simulink model "SimulationEchantillinnesClampingMCC_FixedPt"  (R2018b)
settings: Solver=VariableStepAuto  StartTime=0.0  StopTime=2  MaxStep=Ts_elec  RelTol=1e-3
values from neighbouring files (symbols this model uses):
  Cl = 0    [DataMCCEchant.m]
  Imax = Inom    (= 4.4)    [DataMCCEchant.m]
  Imin = 0    [DataMCCEchant.m]
  Kelec = -place(Ae,Be,Pole_elec_desiree)    [DataMCCEchant.m]
  Kmeca = place(Am,Bm,Pole_meca_desiree)    [DataMCCEchant.m]
  Kphi = 0.061    [DataMCCEchant.m]
  Ommax = Omnom    (= 350)    [DataMCCEchant.m]
  Vmax = Vdc    (= 24)    [DataMCCEchant.m]
undefined symbols (not defined in the file or in its folder): DiscIntNeverNeededParam, Ts
libraries: simulink x1
settings Model: Creator=romaindelpoux  LastModifiedBy=Lubin Kerhuel
settings SolverCC: ZeroCrossControl=DisableAll  AlgebraicLoopSolver=LineSearch
settings SFSimCC: SimUseLocalCustomCode=off
settings RTWCC: RTWUseLocalCustomCode=off

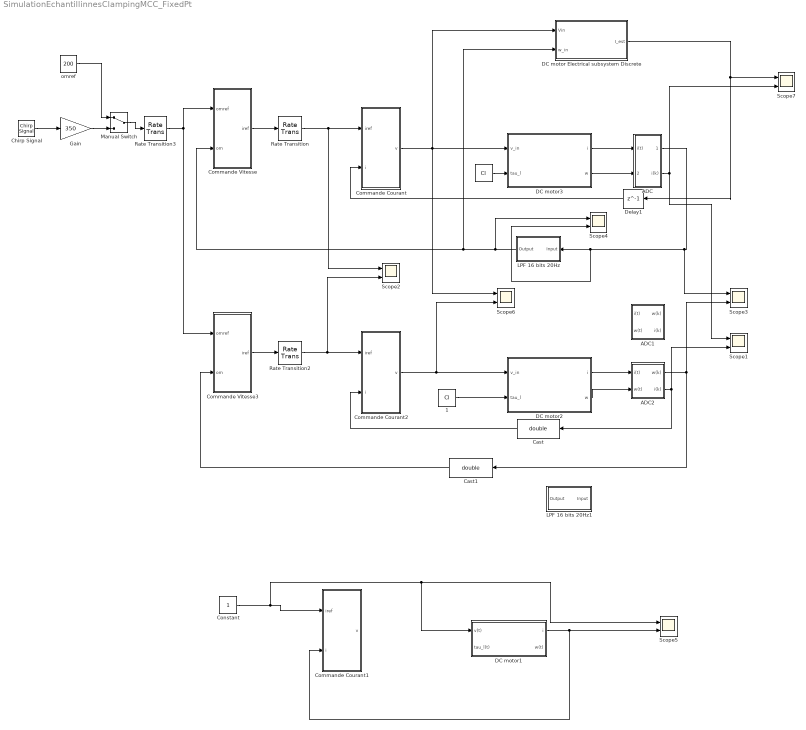
== system SimulationEchantillinnesClampingMCC_FixedPt ==
  " " : Constant  Value=Cl  OutDataTypeStr=Inherit: Inherit via back propagation
  " 1" : Constant  Value=Cl
  ADC : Subsystem
  ADC1 : Subsystem
  ADC2 : Subsystem
  Cast : DataTypeConversion  OutDataTypeStr=double
  Cast1 : DataTypeConversion  OutDataTypeStr=double
  Chirp Signal : simulink/Sources/Chirp Signal  f1=0.1  T=20  f2=5
  Commande Courant : Subsystem
  Commande Courant1 : Subsystem
  Commande Courant2 : Subsystem
  Commande Vitesse : Subsystem
  Commande Vitesse3 : Subsystem
  Constant : Constant
  DC motor Electrical subsystem Discrete : Subsystem
  DC motor1 : Subsystem  mask{R=1.22, L=0.0027, Kphi=0.061, J=0.22e-3, F=.0001, C0=0}
      mask prompts: R "Resistance (R) in Ohms"; L "Inductance (L) in H"; Kphi "Back EMF (Kphi) in V/rad/s"; J "J in kgm²"; F "F in N/rad/s"
      mask DialogControl Container3 Prompt: Electrical Parameters
      mask DialogControl Container3_copy Prompt: Mechanical Parameters
  DC motor2 : Subsystem  mask(Motor PRAVALUX MPM4-0002){R=1.22, L=0.0027, Kphi=0.061, J=0.22e-3, F=.0001, C0=-0.032, mod=0.25}
      mask prompts: R "Resistance (R) in Ohms"; L "Inductance (L) in H"; Kphi "Back EMF (Kphi) in V/rad/s"; J "J in kgm²"; F "F in N/rad/s"; mod "BEMF modulation (default: 0.25, 0 for off)"
      mask help:
      | Continuous time Model for PRAVALUX MPM4 DC motor
      | Caracteristics: 24V DC, 90W, 5.2A, 3000RPM
      |
      | It is a 2nd order model made of two intertwinned system:
      | one 1st order electrical system and one 1st order mechanical system.
      |
      | Modulation on the BEMF can be added to fit with motor current ripple measured
      |
      | Look under mask (Ctrl-U) to see the model
      mask DialogControl Container11 Prompt: Motor
      mask DialogControl Container3 Prompt: Electrical Parameters
      mask DialogControl Container3_copy Prompt: Mechanical Parameters
      mask DialogControl Container14 Prompt: BEMF modulation
      mask Display:
      | color('green');
      | image('MotorPravalux.png');
      | %port_label('input',1,'DC');
      | %port_label('output',1,'BEMF');
  DC motor3 : Subsystem  mask(Motor PRAVALUX MPM4-0002){R=1.22, L=0.0027, Kphi=0.061, J=0.22e-3, F=.0001, C0=-0.032, mod=0.25*0}
      mask prompts: R "Resistance (R) in Ohms"; L "Inductance (L) in H"; Kphi "Back EMF (Kphi) in V/rad/s"; J "J in kgm²"; F "F in N/rad/s"; mod "BEMF modulation (default: 0.25, 0 for off)"
      mask help:
      | Continuous time Model for PRAVALUX MPM4 DC motor
      | Caracteristics: 24V DC, 90W, 5.2A, 3000RPM
      |
      | It is a 2nd order model made of two intertwinned system:
      | one 1st order electrical system and one 1st order mechanical system.
      |
      | Modulation on the BEMF can be added to fit with motor current ripple measured
      |
      | Look under mask (Ctrl-U) to see the model
      mask DialogControl Container11 Prompt: Motor
      mask DialogControl Container3 Prompt: Electrical Parameters
      mask DialogControl Container3_copy Prompt: Mechanical Parameters
      mask DialogControl Container14 Prompt: BEMF modulation
      mask Display:
      | color('green');
      | image('MotorPravalux.png');
      | %port_label('input',1,'DC');
      | %port_label('output',1,'BEMF');
  Delay1 : Delay  DelayLength=1  InitialCondition=0  SampleTime=50e-6
  Gain : Gain  Gain=350  OutDataTypeStr=Inherit: Inherit via back propagation
  LPF 16 bits 20Hz : Subsystem  Tag=FilterWizardSubSystem
      settings: ErrorFcn=dspFilterRealizedInBasicElemsAlgLoopErrFcnCallback
  LPF 16 bits 20Hz1 : Subsystem  Tag=FilterWizardSubSystem
      settings: ErrorFcn=dspFilterRealizedInBasicElemsAlgLoopErrFcnCallback
  Manual Switch : ManualSwitch
  Rate Transition : RateTransition  Deterministic=off  OutPortSampleTime=50e-6
  Rate Transition2 : RateTransition  Deterministic=off  OutPortSampleTime=50e-6
  Rate Transition3 : RateTransition  Deterministic=off  OutPortSampleTime=.002
  Scope{1..7} (7 alike) : Scope  NumInputPorts=2
  omref : Constant  Value=200  OutDataTypeStr=Inherit: Inherit via back propagation
  wires:
  Commande Vitesse/1(iref) -> Rate Transition/1
  DC motor3/1(i) -> ADC/1(i(t))
  DC motor3/2(w) -> ADC/2(w(t))
  ADC/2(i(k)) -> Scope7/2, Scope1/1
  Commande Courant/1(v) -> DC motor Electrical subsystem Discrete/1(Vin), Scope6/1, DC motor3/1(v_in)
  Chirp Signal/1 -> Gain/1
  Rate Transition/1 -> Commande Courant/1(iref), Scope2/1
  DC motor2/2(w) -> ADC2/2(w(t))
  ADC2/2(i(k)) -> Scope1/2, Cast/1
  " 1"/1 -> DC motor2/2(tau_l)
  Commande Vitesse3/1(iref) -> Rate Transition2/1
  Commande Courant2/1(v) -> Scope6/2, DC motor2/1(v_in)
  Rate Transition3/1 -> Commande Vitesse3/1(omref), Commande Vitesse/1(omref)
  Gain/1 -> Manual Switch/2
  Manual Switch/1 -> Rate Transition3/1
  omref/1 -> Manual Switch/1
  ADC/1(w(k)) -> Scope3/1, Scope4/2, LPF 16 bits 20Hz/1(Input)
  Rate Transition2/1 -> Scope2/2, Commande Courant2/1(iref)
  Cast/1 -> Commande Courant2/2(i)
  Cast1/1 -> Commande Vitesse3/2(om)
  LPF 16 bits 20Hz/1(Output) -> Scope4/1, DC motor Electrical subsystem Discrete/2(w_in), Commande Vitesse/2(om)
  ADC2/1(w(k)) -> Cast1/1, Scope3/2
  Constant/1 -> DC motor1/1(v(t)), Scope5/1, Commande Courant1/1(iref)
  DC motor1/1(i) -> Scope5/2, Commande Courant1/2(i)
  " "/1 -> DC motor3/2(tau_l)
  DC motor2/1(i) -> ADC2/1(i(t))
  Delay1/1 -> Commande Courant/2(i)
  DC motor Electrical subsystem Discrete/1(I_est) -> Delay1/1, Scope7/1

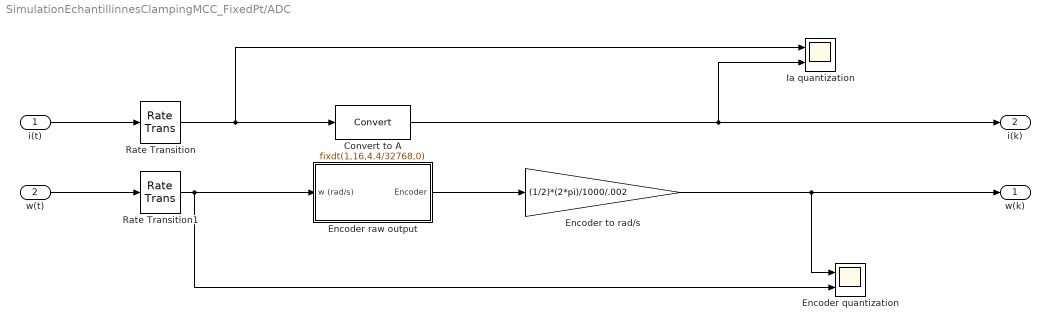
== system SimulationEchantillinnesClampingMCC_FixedPt/ADC ==
  i(t) : Inport
  w(t) : Inport  Port=2
  Convert to A : DataTypeConversion  OutDataTypeStr=fixdt(1,16,4.4/32768,0)  SaturateOnIntegerOverflow=on  LockScale=on
  Encoder quantization : Scope  NumInputPorts=2
  Encoder raw output : Subsystem
  Encoder to rad/s : Gain  Gain=(1/2)*(2*pi)/1000/.002  OutMax=Ommax  OutDataTypeStr=fixdt(1,16)  LockScale=on
  Ia quantization : Scope  NumInputPorts=2
  Rate Transition : RateTransition  Deterministic=off  OutPortSampleTime=.00005
  Rate Transition1 : RateTransition  Deterministic=off  OutPortSampleTime=.002
  w(k) : Outport
  i(k) : Outport  Port=2
  wires:
  Rate Transition/1 -> Ia quantization/1, Convert to A/1
  i(t)/1 -> Rate Transition/1
  w(t)/1 -> Rate Transition1/1
  Encoder to rad/s/1 -> w(k)/1, Encoder quantization/1
  Convert to A/1 -> Ia quantization/2, i(k)/1
  Rate Transition1/1 -> Encoder raw output/1(w (rad/s)), Encoder quantization/2
  Encoder raw output/1(Encoder) -> Encoder to rad/s/1

== system SimulationEchantillinnesClampingMCC_FixedPt/ADC1 ==
  i(t) : Inport
  w(t) : Inport  Port=2
  Rate Transition : RateTransition  Deterministic=off  OutPortSampleTime=50e-6
  Rate Transition1 : RateTransition  Deterministic=off  OutPortSampleTime=.002
  w(k) : Outport
  i(k) : Outport  Port=2
  wires:
  w(t)/1 -> Rate Transition1/1
  i(t)/1 -> Rate Transition/1
  Rate Transition1/1 -> w(k)/1
  Rate Transition/1 -> i(k)/1

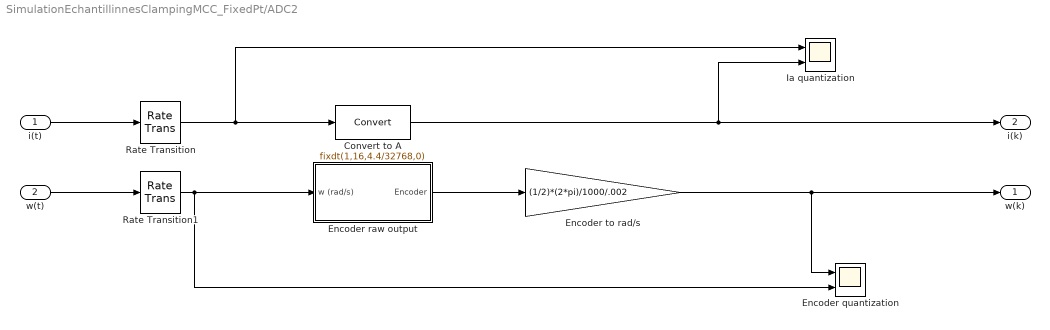
== system SimulationEchantillinnesClampingMCC_FixedPt/ADC2 ==
  i(t) : Inport
  w(t) : Inport  Port=2
  Convert to A : DataTypeConversion  OutDataTypeStr=fixdt(1,16,4.4/32768,0)  SaturateOnIntegerOverflow=on  LockScale=on
  Encoder quantization : Scope  NumInputPorts=2
  Encoder raw output : Subsystem
  Encoder to rad/s : Gain  Gain=(1/2)*(2*pi)/1000/.002  OutMax=Ommax  OutDataTypeStr=fixdt(1,16)  LockScale=on
  Ia quantization : Scope  NumInputPorts=2
  Rate Transition : RateTransition  Deterministic=off  OutPortSampleTime=.00005
  Rate Transition1 : RateTransition  Deterministic=off  OutPortSampleTime=.002
  w(k) : Outport
  i(k) : Outport  Port=2
  wires:
  Encoder raw output/1(Encoder) -> Encoder to rad/s/1
  Rate Transition1/1 -> Encoder quantization/2, Encoder raw output/1(w (rad/s))
  Convert to A/1 -> i(k)/1, Ia quantization/2
  Encoder to rad/s/1 -> Encoder quantization/1, w(k)/1
  w(t)/1 -> Rate Transition1/1
  i(t)/1 -> Rate Transition/1
  Rate Transition/1 -> Convert to A/1, Ia quantization/1

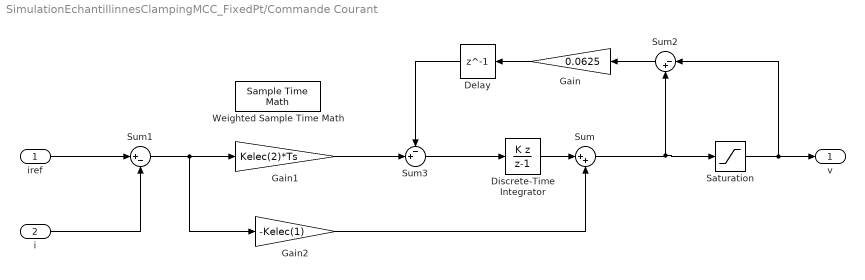
== system SimulationEchantillinnesClampingMCC_FixedPt/Commande Courant ==
  iref : Inport
  i : Inport  Port=2
  Delay : Delay  DelayLength=1  InitialCondition=0
  Discrete-Time Integrator : DiscreteIntegrator  IntegratorMethod=Accumulation: Backward Euler  SampleTime=.00005  OutMax=Vmax*2  OutDataTypeStr=fixdt(1,32)  SaturateOnIntegerOverflow=on  ICPrevOutput=DiscIntNeverNeededParam  ICPrevScaledInput=DiscIntNeverNeededParam
  Gain : Gain  Gain=0.0625  OutDataTypeStr=Inherit: Inherit via back propagation  SaturateOnIntegerOverflow=on
  Gain1 : Gain  Gain=Kelec(2)*Ts  OutMax=2*Imax*Kelec(2)*Ts  OutDataTypeStr=fixdt(1,16)  SaturateOnIntegerOverflow=on
  Gain2 : Gain  Gain=-Kelec(1)  OutMax=Vmax  OutDataTypeStr=fixdt(1,16)  SaturateOnIntegerOverflow=on
  Saturation : Saturate  UpperLimit=Vmax  LowerLimit=-Vmax
  Sum : Sum  Inputs=|++  OutMax=Vmax*2  OutDataTypeStr=fixdt(1,16)  SaturateOnIntegerOverflow=on
  Sum1 : Sum  Inputs=|+-  OutDataTypeStr=fixdt(1,16,12)  SaturateOnIntegerOverflow=on
  Sum2 : Sum  Inputs=|-+  OutDataTypeStr=Inherit: Same as first input
  Sum3 : Sum  Inputs=-+|  OutDataTypeStr=Inherit: Same as accumulator  SaturateOnIntegerOverflow=on  InputSameDT=on
  Weighted Sample Time Math : SampleTimeMath  TsampMathOp=*  weightValue=Kelec(2)  TsampMathImp=Offline Scaling Adjustment
  v : Outport
  wires:
  iref/1 -> Sum1/1
  i/1 -> Sum1/2
  Sum1/1 -> Gain1/1, Gain2/1
  Gain1/1 -> Sum3/2
  Gain2/1 -> Sum/2
  Sum/1 -> Saturation/1, Sum2/2
  Saturation/1 -> v/1, Sum2/1
  Discrete-Time Integrator/1 -> Sum/1
  Sum3/1 -> Discrete-Time Integrator/1
  Sum2/1 -> Gain/1
  Gain/1 -> Delay/1
  Delay/1 -> Sum3/1

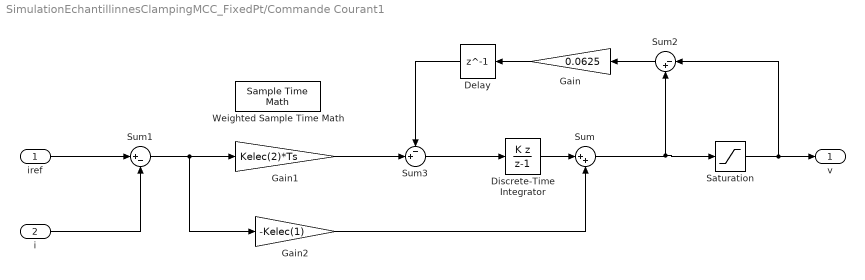
== system SimulationEchantillinnesClampingMCC_FixedPt/Commande Courant1 ==
  iref : Inport
  i : Inport  Port=2
  Delay : Delay  DelayLength=1  InitialCondition=0
  Discrete-Time Integrator : DiscreteIntegrator  IntegratorMethod=Accumulation: Backward Euler  SampleTime=.00005  OutMax=Vmax*2  OutDataTypeStr=fixdt(1,32)  SaturateOnIntegerOverflow=on  ICPrevOutput=DiscIntNeverNeededParam  ICPrevScaledInput=DiscIntNeverNeededParam
  Gain : Gain  Gain=0.0625  OutDataTypeStr=Inherit: Inherit via back propagation  SaturateOnIntegerOverflow=on
  Gain1 : Gain  Gain=Kelec(2)*Ts  OutMax=2*Imax*Kelec(2)*Ts  OutDataTypeStr=fixdt(1,16)  SaturateOnIntegerOverflow=on
  Gain2 : Gain  Gain=-Kelec(1)  OutMax=Vmax  OutDataTypeStr=fixdt(1,16)  SaturateOnIntegerOverflow=on
  Saturation : Saturate  UpperLimit=Vmax  LowerLimit=-Vmax
  Sum : Sum  Inputs=|++  OutMax=Vmax*2  OutDataTypeStr=fixdt(1,16)  SaturateOnIntegerOverflow=on
  Sum1 : Sum  Inputs=|+-  OutDataTypeStr=fixdt(1,16,12)  SaturateOnIntegerOverflow=on
  Sum2 : Sum  Inputs=|-+  OutDataTypeStr=Inherit: Same as first input
  Sum3 : Sum  Inputs=-+|  OutDataTypeStr=Inherit: Same as accumulator  SaturateOnIntegerOverflow=on  InputSameDT=on
  Weighted Sample Time Math : SampleTimeMath  TsampMathOp=*  weightValue=Kelec(2)  TsampMathImp=Offline Scaling Adjustment
  v : Outport
  wires:
  Delay/1 -> Sum3/1
  Gain/1 -> Delay/1
  Sum2/1 -> Gain/1
  Sum3/1 -> Discrete-Time Integrator/1
  Discrete-Time Integrator/1 -> Sum/1
  Saturation/1 -> Sum2/1, v/1
  Sum/1 -> Sum2/2, Saturation/1
  Gain2/1 -> Sum/2
  Gain1/1 -> Sum3/2
  Sum1/1 -> Gain2/1, Gain1/1
  i/1 -> Sum1/2
  iref/1 -> Sum1/1

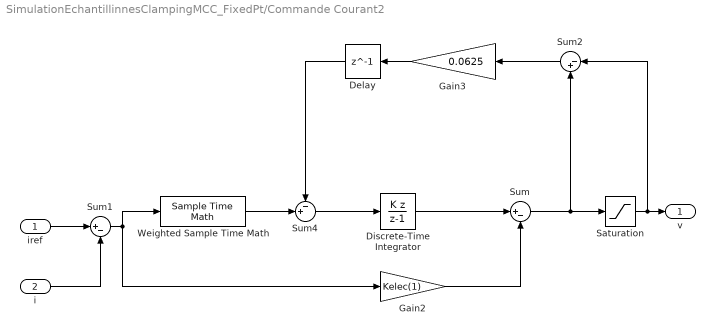
== system SimulationEchantillinnesClampingMCC_FixedPt/Commande Courant2 ==
  iref : Inport
  i : Inport  Port=2
  Delay : Delay  DelayLength=1  InitialCondition=0
  Discrete-Time Integrator : DiscreteIntegrator  IntegratorMethod=Accumulation: Backward Euler  SampleTime=-1  ICPrevOutput=DiscIntNeverNeededParam  ICPrevScaledInput=DiscIntNeverNeededParam
  Gain2 : Gain  Gain=Kelec(1)
  Gain3 : Gain  Gain=0.0625
  Saturation : Saturate  UpperLimit=Vmax  LowerLimit=-Vmax
  Sum : Sum  Inputs=|+-
  Sum1 : Sum  Inputs=|+-
  Sum2 : Sum  Inputs=|-+  OutDataTypeStr=Inherit: Same as accumulator
  Sum4 : Sum  Inputs=-+|
  Weighted Sample Time Math : SampleTimeMath  TsampMathOp=*  weightValue=Kelec(2)  TsampMathImp=Offline Scaling Adjustment
  v : Outport
  wires:
  Weighted Sample Time Math/1 -> Sum4/2
  Sum2/1 -> Gain3/1
  Discrete-Time Integrator/1 -> Sum/1
  Delay/1 -> Sum4/1
  Gain3/1 -> Delay/1
  Sum4/1 -> Discrete-Time Integrator/1
  Sum1/1 -> Weighted Sample Time Math/1, Gain2/1
  Gain2/1 -> Sum/2
  i/1 -> Sum1/2
  iref/1 -> Sum1/1
  Sum/1 -> Sum2/2, Saturation/1
  Saturation/1 -> Sum2/1, v/1

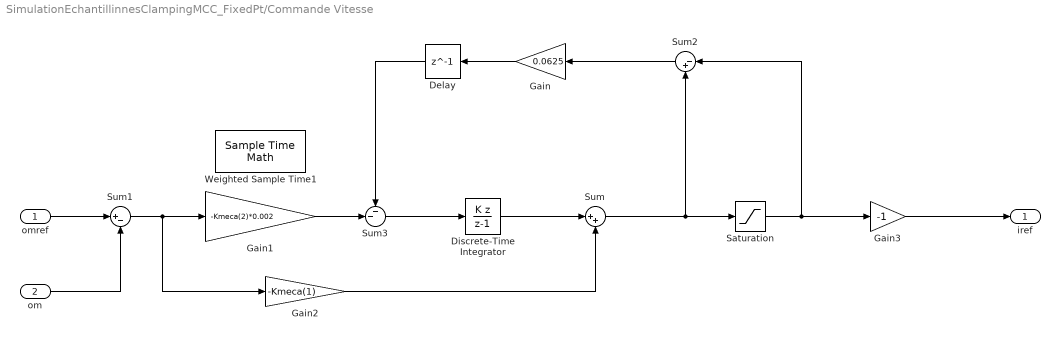
== system SimulationEchantillinnesClampingMCC_FixedPt/Commande Vitesse ==
  omref : Inport  OutMax=[Ommax]  OutDataTypeStr=fixdt(1,16)
  om : Inport  Port=2
  Delay : Delay  DelayLength=1  InitialCondition=0
  Discrete-Time Integrator : DiscreteIntegrator  IntegratorMethod=Accumulation: Backward Euler  SampleTime=.002  OutMin=0  OutMax=Imax*2  OutDataTypeStr=fixdt(1,32)  SaturateOnIntegerOverflow=on  ICPrevOutput=DiscIntNeverNeededParam  ICPrevScaledInput=DiscIntNeverNeededParam
  Gain : Gain  Gain=0.0625  OutDataTypeStr=Inherit: Inherit via back propagation  SaturateOnIntegerOverflow=on
  Gain1 : Gain  Gain=-Kmeca(2)*0.002  OutMin=0  OutMax=abs(Ommax * Kmeca(2) * 0.002)  OutDataTypeStr=fixdt(1,16)
  Gain2 : Gain  Gain=-Kmeca(1)  OutMin=Imin*2  OutMax=Imax*2  OutDataTypeStr=fixdt(1,16)  SaturateOnIntegerOverflow=on
  Gain3 : Gain  Gain=-1  OutMin=Imin  OutMax=Imax  SaturateOnIntegerOverflow=on  OutDataTypeStr=Inherit: Same as input
  Saturation : Saturate  UpperLimit=Imax  LowerLimit=-Imax
  Sum : Sum  Inputs=|++  OutMin=Imin  OutMax=Imax*2  OutDataTypeStr=fixdt(1,16)  SaturateOnIntegerOverflow=on
  Sum1 : Sum  Inputs=|+-  OutMin=-Ommax*2  OutMax=Ommax*2  OutDataTypeStr=fixdt(1,16)
  Sum2 : Sum  Inputs=|-+  OutDataTypeStr=Inherit: Same as accumulator
  Sum3 : Sum  Inputs=--|  OutDataTypeStr=Inherit: Same as accumulator  SaturateOnIntegerOverflow=on  InputSameDT=on
  Weighted Sample Time1 : SampleTimeMath  TsampMathOp=*  weightValue=-Kmeca(2)  TsampMathImp=Offline Scaling Adjustment
  iref : Outport
  wires:
  omref/1 -> Sum1/1
  Gain2/1 -> Sum/2
  om/1 -> Sum1/2
  Sum/1 -> Sum2/2, Saturation/1
  Saturation/1 -> Sum2/1, Gain3/1
  Sum3/1 -> Discrete-Time Integrator/1
  Sum2/1 -> Gain/1
  Gain3/1 -> iref/1
  Sum1/1 -> Gain1/1, Gain2/1
  Gain/1 -> Delay/1
  Delay/1 -> Sum3/1
  Discrete-Time Integrator/1 -> Sum/1
  Gain1/1 -> Sum3/2

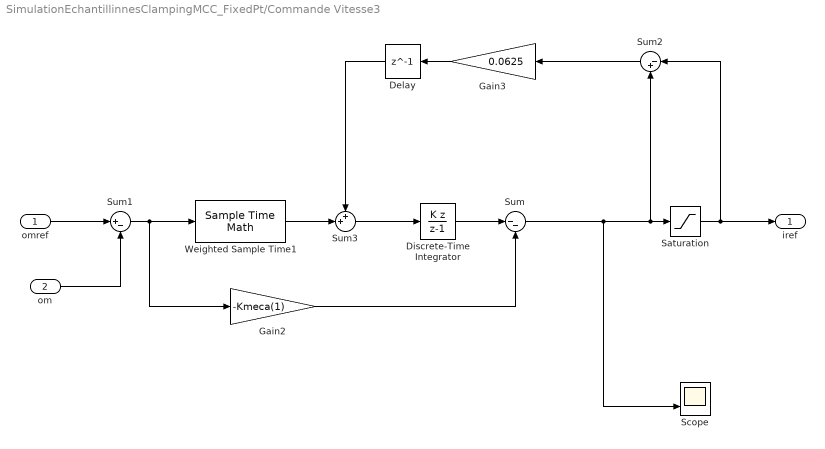
== system SimulationEchantillinnesClampingMCC_FixedPt/Commande Vitesse3 ==
  omref : Inport
  om : Inport  Port=2
  Delay : Delay  DelayLength=1  InitialCondition=0
  Discrete-Time Integrator : DiscreteIntegrator  IntegratorMethod=Accumulation: Backward Euler  SampleTime=-1  ICPrevOutput=DiscIntNeverNeededParam  ICPrevScaledInput=DiscIntNeverNeededParam
  Gain2 : Gain  Gain=-Kmeca(1)
  Gain3 : Gain  Gain=0.0625  OutDataTypeStr=Inherit: Inherit via back propagation
  Saturation : Saturate  UpperLimit=Imax  LowerLimit=-Imax
  Scope : Scope  NumInputPorts=2
  Sum : Sum  Inputs=|--
  Sum1 : Sum  Inputs=|+-
  Sum2 : Sum  Inputs=|-+  OutDataTypeStr=Inherit: Same as accumulator
  Sum3 : Sum  Inputs=++|
  Weighted Sample Time1 : SampleTimeMath  TsampMathOp=*  weightValue=Kmeca(2)
  iref : Outport
  wires:
  Gain2/1 -> Sum/2
  Sum2/1 -> Gain3/1
  Sum1/1 -> Weighted Sample Time1/1, Gain2/1
  omref/1 -> Sum1/1
  om/1 -> Sum1/2
  Sum/1 -> Saturation/1, Sum2/2, Scope/2
  Saturation/1 -> Sum2/1, iref/1
  Discrete-Time Integrator/1 -> Sum/1
  Sum3/1 -> Discrete-Time Integrator/1
  Weighted Sample Time1/1 -> Sum3/2
  Gain3/1 -> Delay/1
  Delay/1 -> Sum3/1

== system SimulationEchantillinnesClampingMCC_FixedPt/DC motor Electrical subsystem Discrete ==
  note: Discrete model of Electrical system:
      | sys_elec = tf(1/R,[L/R 1]);
      | sys_elecz = c2d(sys_elec,50e-6,'zoh')
      |
      | To be used as internal model
  Vin : Inport
  w_in : Inport  Port=2
  Delay : Delay  DelayLength=1  InitialCondition=0  SampleTime=50e-6
  Gain1 : Gain  Gain=-0.977  OutDataTypeStr=fixdt(1,32,9)  SaturateOnIntegerOverflow=on
  Gain3 : Gain  Gain=0.0183  OutMin=[-8.8]  OutMax=8.8  OutDataTypeStr=fixdt(1,16)  SaturateOnIntegerOverflow=on
  Gain4 : Gain  Gain=Kphi  OutDataTypeStr=Inherit: Inherit via back propagation  SaturateOnIntegerOverflow=on
  Rate Transition1 : RateTransition  Deterministic=off  OutPortSampleTime=50e-6
  Sum2 : Sum  Inputs=+--  SaturateOnIntegerOverflow=on
  I_est : Outport
  wires:
  Gain3/1 -> I_est/1
  w_in/1 -> Rate Transition1/1
  Sum2/1 -> Delay/1, Gain3/1
  Gain4/1 -> Sum2/2
  Gain1/1 -> Sum2/3
  Rate Transition1/1 -> Gain4/1
  Vin/1 -> Sum2/1
  Delay/1 -> Gain1/1

== system SimulationEchantillinnesClampingMCC_FixedPt/DC motor1 ==
  v(t) : Inport
  tau_l(t) : Inport  Port=2
  Equation Electrique : Subsystem
  Equation Mecanique : Subsystem
  Gain1 : Gain  Gain=Kphi
  "Gain3  " : Gain  Gain=Kphi
  i : Outport
  w(t) : Outport  Port=2
  wires:
  Gain1/1 -> Equation Mecanique/1(C)
  tau_l(t)/1 -> Equation Mecanique/2(Cl)
  Equation Electrique/1(i(t)) -> i/1, Gain1/1
  Equation Mecanique/1(omega) -> w(t)/1, "Gain3  "/1
  v(t)/1 -> Equation Electrique/1(v)

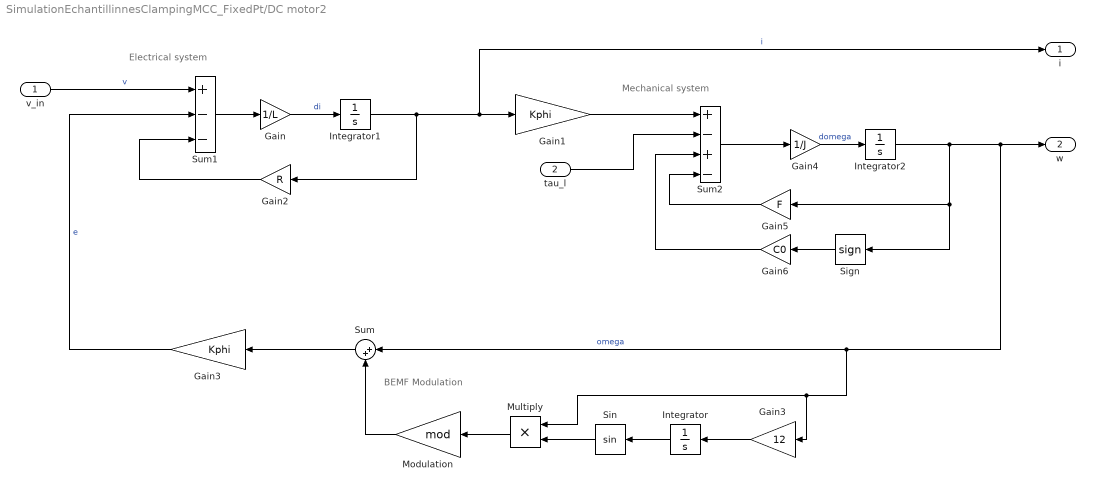
== system SimulationEchantillinnesClampingMCC_FixedPt/DC motor2 ==
  note: BEMF Modulation
  note: Mechanical system
  note: Electrical system
  v_in : Inport  SampleTime=0
  tau_l : Inport  Port=2
  Gain : Gain  Gain=1/L
  Gain1 : Gain  Gain=Kphi
  Gain2 : Gain  Gain=R
  Gain3 : Gain  Gain=12
  "Gain3  " : Gain  Gain=Kphi
  Gain4 : Gain  Gain=1/J
  Gain5 : Gain  Gain=F
  Gain6 : Gain  Gain=C0
  Integrator : Integrator  WrapState=on
  Integrator1 : Integrator
  Integrator2 : Integrator
  Modulation : Gain  Gain=mod
  Multiply : Product
  Sign : Signum
  Sin : Trigonometry
  Sum : Sum  Inputs=|++
  Sum1 : Sum  Inputs=+--
  Sum2 : Sum  Inputs=+-+-
  i : Outport
  w : Outport  Port=2
  wires:
  Sin/1 -> Multiply/2
  Sum/1 -> "Gain3  "/1
  Modulation/1 -> Sum/2
  Multiply/1 -> Modulation/1
  Integrator/1 -> Sin/1
  Gain3/1 -> Integrator/1
  Sum1/1 -> Gain/1
  Gain/1 -> Integrator1/1  "di"
  Integrator1/1 -> Gain2/1, i/1, Gain1/1  "i"
  v_in/1 -> Sum1/1  "v"
  Gain2/1 -> Sum1/3
  "Gain3  "/1 -> Sum1/2  "e"
  tau_l/1 -> Sum2/2
  Gain6/1 -> Sum2/3
  Sign/1 -> Gain6/1
  Integrator2/1 -> w/1, Sum/1, Gain3/1, Multiply/1, Sign/1, Gain5/1  "omega"
  Gain5/1 -> Sum2/4
  Sum2/1 -> Gain4/1
  Gain4/1 -> Integrator2/1  "domega"
  Gain1/1 -> Sum2/1

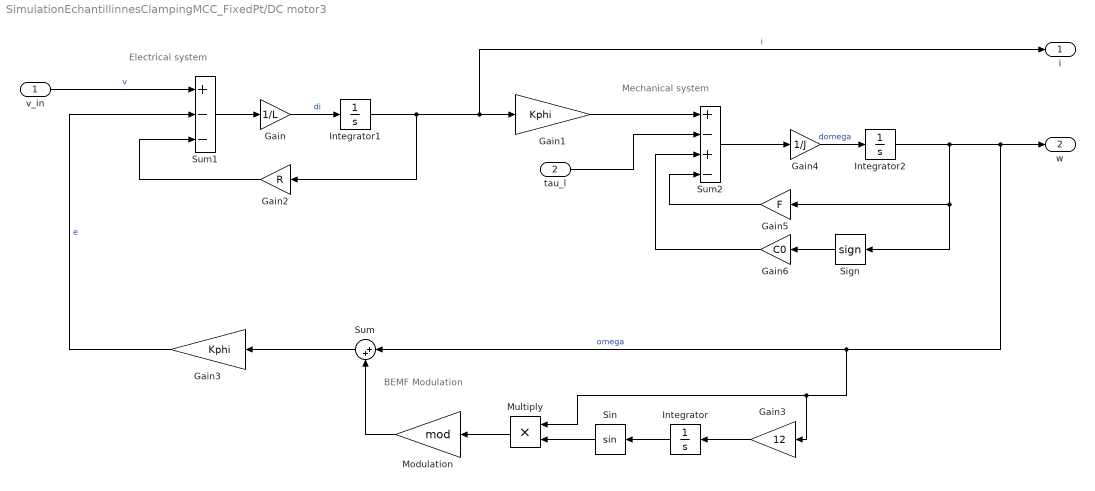
== system SimulationEchantillinnesClampingMCC_FixedPt/DC motor3 ==
  note: Electrical system
  note: Mechanical system
  note: BEMF Modulation
  v_in : Inport  SampleTime=0
  tau_l : Inport  Port=2
  Gain : Gain  Gain=1/L
  Gain1 : Gain  Gain=Kphi
  Gain2 : Gain  Gain=R
  Gain3 : Gain  Gain=12
  "Gain3  " : Gain  Gain=Kphi
  Gain4 : Gain  Gain=1/J
  Gain5 : Gain  Gain=F
  Gain6 : Gain  Gain=C0
  Integrator : Integrator  WrapState=on
  Integrator1 : Integrator
  Integrator2 : Integrator
  Modulation : Gain  Gain=mod
  Multiply : Product
  Sign : Signum
  Sin : Trigonometry
  Sum : Sum  Inputs=|++
  Sum1 : Sum  Inputs=+--
  Sum2 : Sum  Inputs=+-+-
  i : Outport
  w : Outport  Port=2
  wires:
  Gain1/1 -> Sum2/1
  Gain4/1 -> Integrator2/1  "domega"
  Sum2/1 -> Gain4/1
  Gain5/1 -> Sum2/4
  Integrator2/1 -> Gain5/1, Sign/1, Multiply/1, Gain3/1, Sum/1, w/1  "omega"
  Sign/1 -> Gain6/1
  Gain6/1 -> Sum2/3
  tau_l/1 -> Sum2/2
  "Gain3  "/1 -> Sum1/2  "e"
  Gain2/1 -> Sum1/3
  v_in/1 -> Sum1/1  "v"
  Integrator1/1 -> Gain1/1, i/1, Gain2/1  "i"
  Gain/1 -> Integrator1/1  "di"
  Sum1/1 -> Gain/1
  Gain3/1 -> Integrator/1
  Integrator/1 -> Sin/1
  Multiply/1 -> Modulation/1
  Modulation/1 -> Sum/2
  Sum/1 -> "Gain3  "/1
  Sin/1 -> Multiply/2

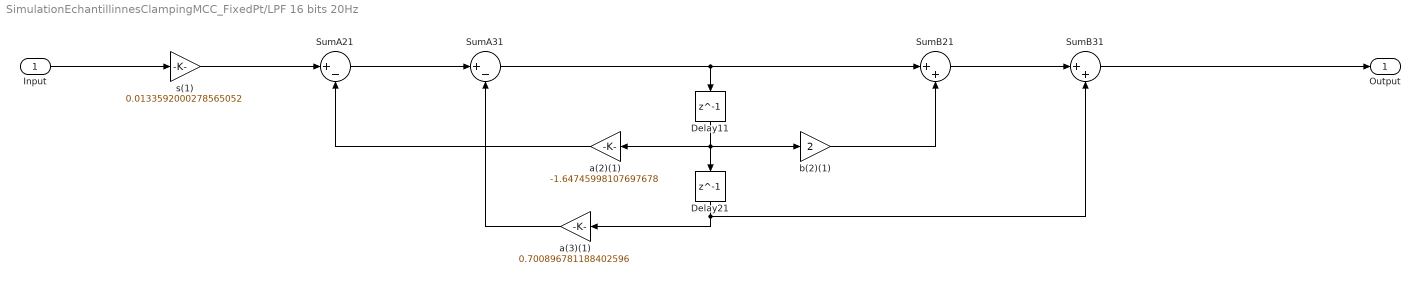
== system SimulationEchantillinnesClampingMCC_FixedPt/LPF 16 bits 20Hz ==
  Input : Inport
  Delay11 : Delay  DelayLength=1  InitialCondition=0
  Delay21 : Delay  DelayLength=1  InitialCondition=0
  SumA21 : Sum  Inputs=|+-  OutDataTypeStr=fixdt(1,16,6)  RndMeth=Nearest  SaturateOnIntegerOverflow=on
  SumA31 : Sum  Inputs=|+-  OutDataTypeStr=fixdt(1,16,6)  RndMeth=Nearest  SaturateOnIntegerOverflow=on
  SumB21 : Sum  Inputs=|++  OutDataTypeStr=fixdt(1,16,5)  RndMeth=Nearest  SaturateOnIntegerOverflow=on
  SumB31 : Sum  Inputs=|++  OutDataTypeStr=fixdt(1,16,4)  RndMeth=Nearest  SaturateOnIntegerOverflow=on
  a(2)(1) : Gain  Gain=-1.64745998107697678  ParamDataTypeStr=fixdt(1,16,14)  OutDataTypeStr=fixdt(1,16,6)  RndMeth=Nearest  SaturateOnIntegerOverflow=on
  a(3)(1) : Gain  Gain=0.700896781188402596  ParamDataTypeStr=fixdt(0,16,16)  OutDataTypeStr=fixdt(1,16,7)  RndMeth=Nearest  SaturateOnIntegerOverflow=on
  b(2)(1) : Gain  Gain=2  ParamDataTypeStr=fixdt(0,16,14)  OutDataTypeStr=fixdt(1,16,5)  RndMeth=Nearest  SaturateOnIntegerOverflow=on
  s(1) : Gain  Gain=0.0133592000278565052  ParamDataTypeStr=fixdt(0,16,22)  OutDataTypeStr=fixdt(1,16,11)  RndMeth=Nearest  SaturateOnIntegerOverflow=on
  Output : Outport
  wires:
  Input/1 -> s(1)/1
  s(1)/1 -> SumA21/1
  SumA21/1 -> SumA31/1
  SumA31/1 -> SumB21/1, Delay11/1
  SumB21/1 -> SumB31/1
  SumB31/1 -> Output/1
  a(2)(1)/1 -> SumA21/2
  Delay11/1 -> a(2)(1)/1, b(2)(1)/1, Delay21/1
  b(2)(1)/1 -> SumB21/2
  a(3)(1)/1 -> SumA31/2
  Delay21/1 -> a(3)(1)/1, SumB31/2

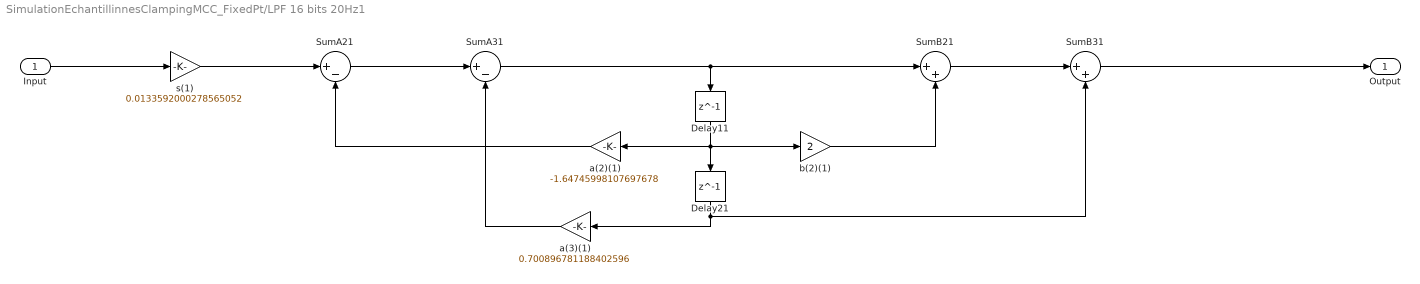
== system SimulationEchantillinnesClampingMCC_FixedPt/LPF 16 bits 20Hz1 ==
  Input : Inport
  Delay11 : Delay  DelayLength=1  InitialCondition=0
  Delay21 : Delay  DelayLength=1  InitialCondition=0
  SumA21 : Sum  Inputs=|+-  OutDataTypeStr=fixdt(1,16,6)  RndMeth=Nearest  SaturateOnIntegerOverflow=on
  SumA31 : Sum  Inputs=|+-  OutDataTypeStr=fixdt(1,16,6)  RndMeth=Nearest  SaturateOnIntegerOverflow=on
  SumB21 : Sum  Inputs=|++  OutDataTypeStr=fixdt(1,16,5)  RndMeth=Nearest  SaturateOnIntegerOverflow=on
  SumB31 : Sum  Inputs=|++  OutDataTypeStr=fixdt(1,16,4)  RndMeth=Nearest  SaturateOnIntegerOverflow=on
  a(2)(1) : Gain  Gain=-1.64745998107697678  ParamDataTypeStr=fixdt(1,16,14)  OutDataTypeStr=fixdt(1,16,6)  RndMeth=Nearest  SaturateOnIntegerOverflow=on
  a(3)(1) : Gain  Gain=0.700896781188402596  ParamDataTypeStr=fixdt(0,16,16)  OutDataTypeStr=fixdt(1,16,7)  RndMeth=Nearest  SaturateOnIntegerOverflow=on
  b(2)(1) : Gain  Gain=2  ParamDataTypeStr=fixdt(0,16,14)  OutDataTypeStr=fixdt(1,16,5)  RndMeth=Nearest  SaturateOnIntegerOverflow=on
  s(1) : Gain  Gain=0.0133592000278565052  ParamDataTypeStr=fixdt(0,16,22)  OutDataTypeStr=fixdt(1,16,11)  RndMeth=Nearest  SaturateOnIntegerOverflow=on
  Output : Outport
  wires:
  Delay21/1 -> SumB31/2, a(3)(1)/1
  a(3)(1)/1 -> SumA31/2
  b(2)(1)/1 -> SumB21/2
  Delay11/1 -> Delay21/1, b(2)(1)/1, a(2)(1)/1
  a(2)(1)/1 -> SumA21/2
  SumB31/1 -> Output/1
  SumB21/1 -> SumB31/1
  SumA31/1 -> Delay11/1, SumB21/1
  SumA21/1 -> SumA31/1
  s(1)/1 -> SumA21/1
  Input/1 -> s(1)/1

== system SimulationEchantillinnesClampingMCC_FixedPt/ADC/Encoder raw output ==
  w (rad/s) : Inport
  Encoder output : DataTypeConversion  OutDataTypeStr=int16  SaturateOnIntegerOverflow=on  LockScale=on
  Gain1 : Gain  Gain="inv(  (1/2)*(2*pi)/1000/.002  )"  OutDataTypeStr=double  LockScale=on
  Encoder : Outport
  wires:
  Gain1/1 -> Encoder output/1
  Encoder output/1 -> Encoder/1
  w (rad/s)/1 -> Gain1/1

== system SimulationEchantillinnesClampingMCC_FixedPt/ADC2/Encoder raw output ==
  w (rad/s) : Inport
  Encoder output : DataTypeConversion  OutDataTypeStr=int16  SaturateOnIntegerOverflow=on  LockScale=on
  Gain1 : Gain  Gain="inv(  (1/2)*(2*pi)/1000/.002  )"  OutDataTypeStr=double  LockScale=on
  Encoder : Outport
  wires:
  w (rad/s)/1 -> Gain1/1
  Encoder output/1 -> Encoder/1
  Gain1/1 -> Encoder output/1

== system SimulationEchantillinnesClampingMCC_FixedPt/DC motor1/Equation Electrique ==
  v : Inport
  e : Inport  Port=2
  Gain : Gain  Gain=1/L
  Gain1 : Gain  Gain=R
  Integrator : Integrator
  Sum : Sum  Inputs=+--
  i(t) : Outport
  wires:
  Gain1/1 -> Sum/2
  Sum/1 -> Gain/1
  Integrator/1 -> i(t)/1, Gain1/1  "i"
  Gain/1 -> Integrator/1  "di"
  v/1 -> Sum/1
  e/1 -> Sum/3

== system SimulationEchantillinnesClampingMCC_FixedPt/DC motor1/Equation Mecanique ==
  C : Inport
  Cl : Inport  Port=2
  Gain : Gain  Gain=1/J
  Gain1 : Gain  Gain=F
  Gain2 : Gain  Gain=C0
  Integrator : Integrator
  Sign : Signum
  Sum : Sum  Inputs=+-+-
  omega : Outport
  wires:
  Gain/1 -> Integrator/1  "domega"
  Integrator/1 -> Sign/1, Gain1/1, omega/1  "omega"
  Sum/1 -> Gain/1
  Gain1/1 -> Sum/2
  Sign/1 -> Gain2/1
  Gain2/1 -> Sum/3
  C/1 -> Sum/1
  Cl/1 -> Sum/4
